simulink model "solarmonitor_stateflow"  (R2019b)
settings: Solver=FixedStepAuto  StartTime=0.0  StopTime=10.0  RelTol=1e-3  EnableMultiTasking=on
libraries: raspberrypilib x2
settings Model: SimulationMode=external  Creator=shogo  LastModifiedBy=shogo
settings SolverCC: PositivePriorityOrder=on
settings OptimizationCC: EnhancedBackFolding=on  PassReuseOutputArgsAs=Individual arguments  ZeroExternalMemoryAtStartup=off  ZeroInternalMemoryAtStartup=off  MaxStackSize=64  OptimizeBlockOrder=speed  DifferentSizesBufferReuse=on  OptimizationCustomize=off  EfficientTunableParamExpr=on
settings DebuggingCC: ParameterTunabilityLossMsg=error
settings HardwareCC: ProdBitPerPointer=32  ProdBitPerSizeT=32  ProdBitPerPtrDiffT=32  ProdLargestAtomicInteger=Long  ProdLargestAtomicFloat=Double  ProdWordSize=32  ProdLongLongMode=on  ProdHWDeviceType=ARM Compatible->ARM Cortex  UseEmbeddedCoderFeatures=off  UseSimulinkCoderFeatures=off
settings RTWCC: SystemTargetFile=ert.tlc  HardwareBoard=Raspberry Pi  TLCOptions="-aInlineSetEventsForThisBaseRateFcn=TLC_FALSE -aSuppressMultiTaskScheduler=TLC_FALSE  -aRateBasedStepFcn=0"  TemplateMakefile=ert_default_tmf  RTWVerbose=off  Toolchain=GNU GCC Raspberry Pi  BuildConfiguration=Faster Runs  IncludeHyperlinkInReport=on
settings CodeAppCC: ForceParamTrailComments=on  OperatorAnnotations=on  SimulinkDataObjDesc=on  SFDataObjDesc=on  MangleLength=10  InsertBlockDesc=on
settings ERTTargetCC: SupportNonInlinedSFcns=on  SupportVariableSizeSignals=on  ExtMode=on  ExtModeTransport=2  ExtModeStaticAlloc=on  ExtModeMexFile=ext_xcp  ExtModeMexArgs='192.168.11.21' 0 17725  ExtModeIntrfLevel=Level2 - Open  ERTSrcFileBannerTemplate=codertarget_code_template.cgt  ERTHdrFileBannerTemplate=codertarget_code_template.cgt  ERTDataSrcFileTemplate=codertarget_code_template.cgt  ERTDataHdrFileTemplate=codertarget_code_template.cgt

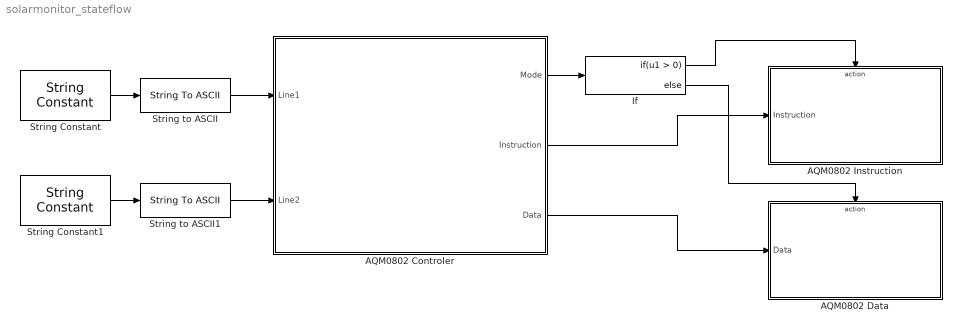
== system solarmonitor_stateflow ==
  AQM0802 Controler : Stateflow chart  BlockKeywords=__PRM__SERIALIZED__DATA__:Stateflow Chart,Stateflow Diagram  TreatAsAtomicUnit=on
  AQM0802 Data : Subsystem  TreatAsAtomicUnit=on
  AQM0802 Instruction : Subsystem  TreatAsAtomicUnit=on
  If : If
  String Constant : StringConstant
  String Constant1 : StringConstant  String="\"World!\""
  String to ASCII : StringToASCII
  String to ASCII1 : StringToASCII
  wires:
  AQM0802 Controler/3(Data) -> AQM0802 Data/1(Data)
  AQM0802 Controler/2(Instruction) -> AQM0802 Instruction/1(Instruction)
  AQM0802 Controler/1(Mode) -> If/1
  If/1 -> AQM0802 Instruction/Action
  If/2 -> AQM0802 Data/Action
  String Constant/1 -> String to ASCII/1
  String Constant1/1 -> String to ASCII1/1
  String to ASCII/1 -> AQM0802 Controler/1(Line1)
  String to ASCII1/1 -> AQM0802 Controler/2(Line2)

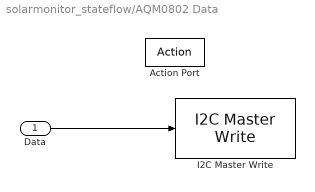
== system solarmonitor_stateflow/AQM0802 Data ==
  Data : Inport
  Action Port : ActionPort  ActionPortLabel=else
  I2C Master Write : raspberrypilib/I2C Master Write  BoardProperty=Pi 3 Model B  Mode=Master  SlaveAddress=0x3e  SlaveByteOrder=BigEndian  Direction=Transmitter  RegisterAddressMode=on  RegisterAddress=0x40  SlaveDataType=uint8  DataLength=1  NoAck=off  RepeatedStart=off  OutputStatus=off
      settings: SourceProductName=Simulink Support Package for Raspberry Pi Hardware  SourceProductBaseCode=RASPPI
  wires:
  Data/1 -> I2C Master Write/1

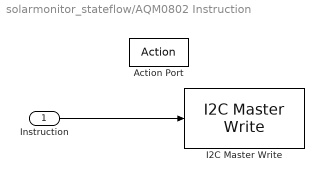
== system solarmonitor_stateflow/AQM0802 Instruction ==
  Instruction : Inport
  Action Port : ActionPort  ActionPortLabel=if(u1 > 0)
  I2C Master Write : raspberrypilib/I2C Master Write  BoardProperty=Pi 3 Model B  Mode=Master  SlaveAddress=0x3e  SlaveByteOrder=BigEndian  Direction=Transmitter  RegisterAddressMode=on  RegisterAddress=0x00  SlaveDataType=uint8  DataLength=1  NoAck=off  RepeatedStart=off  OutputStatus=off
      settings: SourceProductName=Simulink Support Package for Raspberry Pi Hardware  SourceProductBaseCode=RASPPI
  wires:
  Instruction/1 -> I2C Master Write/1

== stateflow chart solarmonitor_stateflow/AQM0802 Controler ==
  state Display_line1
    Mode = 0;
    idx = 1;
    Data = Line1;
  state Initalization
    Mode = 1;
  state Function_set1
    Instruction = 0x38;
  state Move_to_line2
    Mode = 1;
    Instruction = 0xc0;
  state Function_set2
    Instruction = 0x39;
  state Internal_OSC_Freq
    Instruction = 0x14;
  state Display_line2
    Mode = 0;
    idx = 1;
    Data = Line2;
  state Contrast_set
    Instruction = 0x73;
  state PW_ICN_CNT_Ctrl
    Instruction = 0x56;
  state Move_to_line1
    Mode = 1;
    Instruction = 0x80;
  state Follower_Ctrl
    Instruction = 0x6c
  state Function_set3
    Instruction = 0x38;
  state Display_On_Off_Ctrl
    Instruction = 0x0c;
  state Clear_display
    Instruction = 0x01;
  (default) -> Initalization
  Move_to_line1 -> Display_line1
  Initalization -> Function_set1
  Clear_display -> Display_line1 : after(1,msec)
  Display_line1 -> Move_to_line2
  Function_set1 -> Function_set2
  Function_set2 -> Internal_OSC_Freq
  Move_to_line2 -> Display_line2
  Internal_OSC_Freq -> Contrast_set
  Contrast_set -> PW_ICN_CNT_Ctrl
  Display_line2 -> Move_to_line1
  PW_ICN_CNT_Ctrl -> Follower_Ctrl
  Follower_Ctrl -> Function_set3 : after(200,msec)
  Function_set3 -> Display_On_Off_Ctrl
  Display_On_Off_Ctrl -> Clear_display
  data: Mode output; Instruction output; Data output; Line1 input; Line2 input; idx local
